simulink model "delaywithoutdelay"  (R2021a)
settings: Solver=VariableStepAuto  StartTime=0.0  StopTime=10.0  RelTol=1e-3
libraries: simulink x1
settings Model: Creator=surya  LastModifiedBy=surya

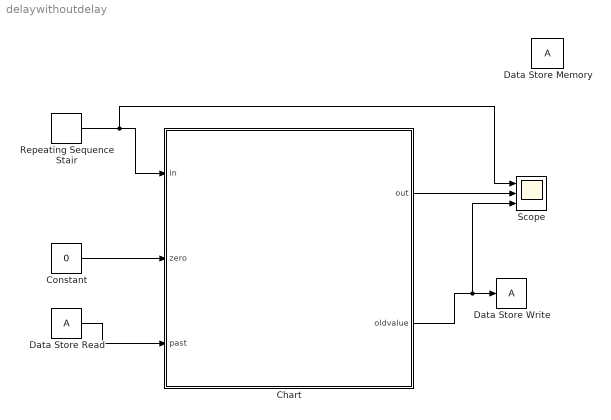
== system delaywithoutdelay ==
  Chart : Stateflow chart  TreatAsAtomicUnit=on
  Constant : Constant  Value=0
  Data Store Memory : DataStoreMemory  ReadBeforeWriteMsg=warning  WriteAfterWriteMsg=warning  WriteAfterReadMsg=warning  ShowAdditionalParam=off
  Data Store Read : DataStoreRead  IndexOptions=Index vector (dialog)  Indices=1  OutputSizes=1
  Data Store Write : DataStoreWrite  IndexOptions=Index vector (dialog)  Indices=1  OutputSizes=1
  Repeating Sequence Stair : simulink/Sources/Repeating Sequence Stair  OutValues=[3 1 4 2 1].'  tsamp=-1  OutMin=[]  OutMax=[]  OutDataTypeStr=double  OutputDataTypeScalingMode=double  OutDataType=fixdt(0,8)  ConRadixGroup=Best Precision: Vector-wise  OutScaling=2^-12
  Scope : Scope  NumInputPorts=3
  wires:
  Data Store Read/1 -> Chart/3(past)
  Repeating Sequence Stair/1 -> Scope/1, Chart/1(in)
  Constant/1 -> Chart/2(zero)
  Chart/2(oldvalue) -> Scope/3, Data Store Write/1
  Chart/1(out) -> Scope/2

== stateflow chart delaywithoutdelay/Chart ==
  (default) -> (junction 7)
  (junction 7) -> (junction 9)
  (junction 9) -> (junction 11) [order 1] : [t==0]{out=zero;
      | oldvalue=in
      | }
  (junction 11) -> (junction 12)
  (junction 9) -> (junction 12) [order 2] : {out=past;
      | oldvalue=in}
  data: out output; in input; zero input; past input; oldvalue output
